simulink model "modelo_dinamico_FL"  (R2024b)
settings: Solver=ode1  StartTime=0.0  StopTime=end_time-Ts  FixedStep=Ts  RelTol=1e-3
undefined symbols (not defined in the file): du1_0, g, k11, k12, k13, k14, k21, k22, k23, k24, k31, k32, k33, k34, k41, k42, lim, M, tau, tau_phi_max, tau_phi_min, tau_psi_max, tau_psi_min, tau_theta_max, tau_theta_min, Ts, u1_0, u_max, u_min, x11_0, x1_0, x3_0, x5_0, x7_0, x9_0
libraries: eeGeneralControl x6, slident x1
settings Model: Creator=pdelr  LastModifiedBy=pdelr
settings DebuggingCC: UnconnectedInputMsg=warning  UnconnectedOutputMsg=warning  UnconnectedLineMsg=warning
settings ModelReferenceCC: EnableRefExpFcnMdlSchedulingChecks=on
settings RTWCC: GPUComputeCapability=3.5  DLArmComputeVersion=19.05

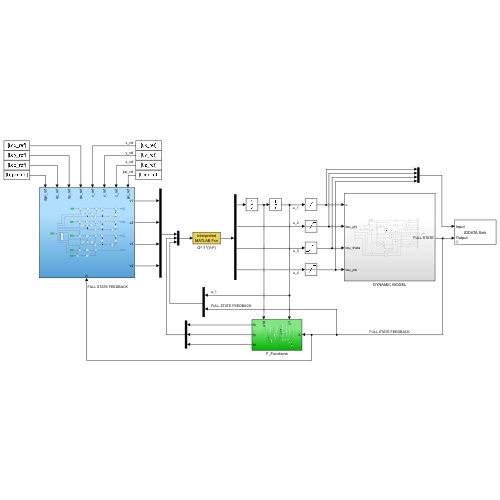
[thumbnail: Simulink's stored preview of the top-level diagram]
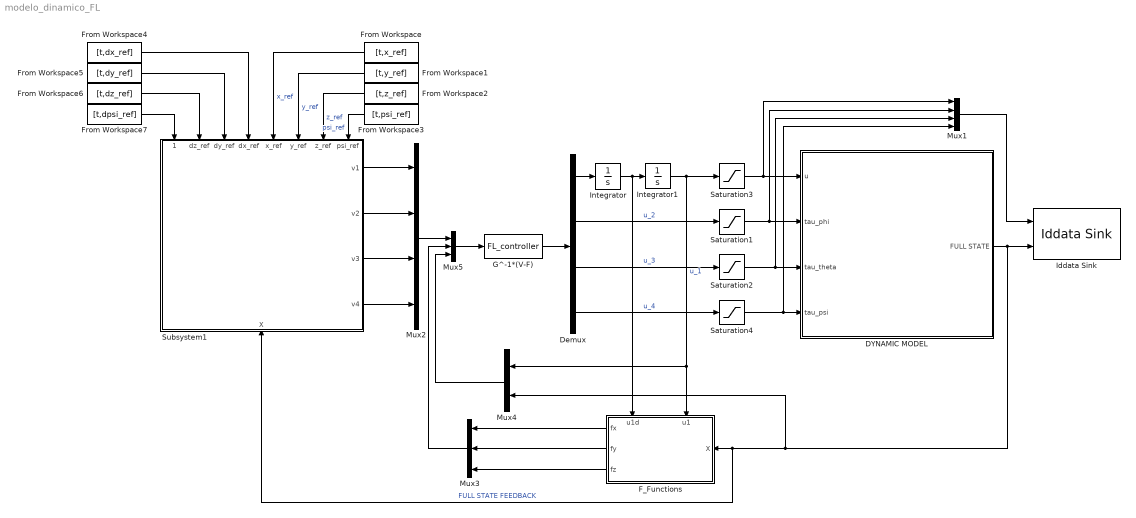
== system modelo_dinamico_FL ==
  DYNAMIC MODEL : Subsystem
  Demux : Demux
  F_Functions : Subsystem
      settings: PortSchema="{\"entries\":[{\"content\":{\"sides\":[{\"content\":{\"connectorIds\":[\"In1\"]},\"type\":\"ConnectorPlacement.EquallySpacedRectSide\",\"uuid\":\"eddb14d5-231a-4b6d-a89c-a6715b5a0e2c\"},{\"content\":{\"connectorIds\":[\"Out1\",\"Out2\",\"Out3\"],\"side\":\"RIGHT\"},\"type\":\"ConnectorPlacement.EquallySpacedRectSide\",\"uuid\":\"e1ae96f0-3fe3-4add-877e-6087d97d73d6\"},{\"content\":{\"connectorIds\":[\"In2\",\"In3\"],\"side\":\"TOP\"},\"type\":\"ConnectorPlacement.EquallySpacedRectSide\",\"uuid\":\"e0d53240-41cb-498f-be06-48178e3678e4\"},{\"content\":{\"connectorIds\":[],\"side\":\"BOTTOM\"},\"type\":\"ConnectorPlacement.EquallySpacedRectSide\",\"uuid\":\"5d003620-640e-4f1b-8c5e-2d3bbf45d64b\"}]},\"type\":\"ConnectorPlacement.EquallySpacedConnector\",\"uuid\":\"d539eae5-8b81-4451-bedc-ec98eec9f474\"}],\"packageUris\":[\"http://schema.mathworks.com/mf0/Connector/R2020b\"],\"version\":\"1.0\"}"
  From Workspace : FromWorkspace  VariableName=[t,x_ref]
  From Workspace1 : FromWorkspace  VariableName=[t,y_ref]
  From Workspace2 : FromWorkspace  VariableName=[t,z_ref]
  From Workspace3 : FromWorkspace  VariableName=[t,psi_ref]
  From Workspace4 : FromWorkspace  VariableName=[t,dx_ref]
  From Workspace5 : FromWorkspace  VariableName=[t,dy_ref]
  From Workspace6 : FromWorkspace  VariableName=[t,dz_ref]
  From Workspace7 : FromWorkspace  VariableName=[t,dpsi_ref]
  G^-1*(V-F) : MATLABFcn  MATLABFcn=FL_controller  OutputDimensions=4
  Iddata Sink : slident/Iddata Sink  datasetname=data  Ts=Ts  isu=off  isy=off
  Integrator : Integrator  InitialCondition=du1_0
  Integrator1 : Integrator  InitialCondition=u1_0  UpperSaturationLimit=lim  LowerSaturationLimit=-lim
  Mux1 : Mux
  Mux2 : Mux
  Mux3 : Mux  Inputs=3
  Mux4 : Mux  Inputs=2
  Mux5 : Mux  Inputs=3
  Saturation1 : Saturate  UpperLimit=tau_phi_max  LowerLimit=tau_phi_min
  Saturation2 : Saturate  UpperLimit=tau_theta_max  LowerLimit=tau_theta_min
  Saturation3 : Saturate  UpperLimit=u_max  LowerLimit=u_min
  Saturation4 : Saturate  UpperLimit=tau_psi_max  LowerLimit=tau_psi_min
  Subsystem1 : Subsystem
      settings: PortSchema="{\"entries\":[{\"content\":{\"sides\":[{\"content\":{\"connectorIds\":[]},\"type\":\"ConnectorPlacement.EquallySpacedRectSide\",\"uuid\":\"eddb14d5-231a-4b6d-a89c-a6715b5a0e2c\"},{\"content\":{\"connectorIds\":[\"Out1\",\"Out2\",\"Out3\",\"Out4\"],\"side\":\"RIGHT\"},\"type\":\"ConnectorPlacement.EquallySpacedRectSide\",\"uuid\":\"e1ae96f0-3fe3-4add-877e-6087d97d73d6\"},{\"content\":{\"connectorIds\":[\"In1\",\"In2\",\"In3\",\"In4\",\"In5\",\"In6\",\"In7\",\"In8\"],\"side\":\"TOP\"},\"type\":\"ConnectorPlacement.EquallySpacedRectSide\",\"uuid\":\"e0d53240-41cb-498f-be06-48178e3678e4\"},{\"content\":{\"connectorIds\":[\"In9\"],\"side\":\"BOTTOM\"},\"type\":\"ConnectorPlacement.EquallySpacedRectSide\",\"uuid\":\"99222e29-004c-4dfd-a165-743ac4cf90b4\"}]},\"type\":\"ConnectorPlacement.EquallySpacedConnector\",\"uuid\":\"d539eae5-8b81-4451-bedc-ec98eec9f474\"}],\"packageUris\":[\"http://schema.mathworks.com/mf0/Connector/R2020b\"],\"version\":\"1.0\"}"
  wires:
  Mux1/1 -> Iddata Sink/1
  Saturation3/1 -> DYNAMIC MODEL/1(u), Mux1/1
  Demux/1 -> Integrator/1
  Integrator1/1 -> Saturation3/1, Mux4/1, F_Functions/2(u1)  "u_1"
  Demux/2 -> Saturation1/1  "u_2"
  Demux/3 -> Saturation2/1  "u_3"
  Demux/4 -> Saturation4/1  "u_4"
  DYNAMIC MODEL/1(FULL STATE) -> Iddata Sink/2, F_Functions/1(X), Subsystem1/9(X), Mux4/2  "FULL STATE FEEDBACK"
  F_Functions/1(fx) -> Mux3/1
  F_Functions/2(fy) -> Mux3/2
  F_Functions/3(fz) -> Mux3/3
  Subsystem1/1(v1) -> Mux2/1
  Subsystem1/2(v2) -> Mux2/2
  Subsystem1/3(v3) -> Mux2/3
  Subsystem1/4(v4) -> Mux2/4
  Mux3/1 -> Mux5/2
  Mux4/1 -> Mux5/3
  Mux2/1 -> Mux5/1
  G^-1*(V-F)/1 -> Demux/1
  From Workspace2/1 -> Subsystem1/7(z_ref)  "z_ref"
  From Workspace3/1 -> Subsystem1/8(psi_ref)  "psi_ref"
  From Workspace/1 -> Subsystem1/5(x_ref)  "x_ref"
  From Workspace1/1 -> Subsystem1/6(y_ref)  "y_ref"
  Mux5/1 -> G^-1*(V-F)/1
  Saturation1/1 -> Mux1/2, DYNAMIC MODEL/2(tau_phi)
  Saturation4/1 -> Mux1/4, DYNAMIC MODEL/4(tau_psi)
  Integrator/1 -> F_Functions/3(u1d), Integrator1/1
  Saturation2/1 -> Mux1/3, DYNAMIC MODEL/3(tau_theta)
  From Workspace4/1 -> Subsystem1/4(dx_ref)
  From Workspace5/1 -> Subsystem1/3(dy_ref)
  From Workspace6/1 -> Subsystem1/2(dz_ref)
  From Workspace7/1 -> Subsystem1/1(dpsi_ref)

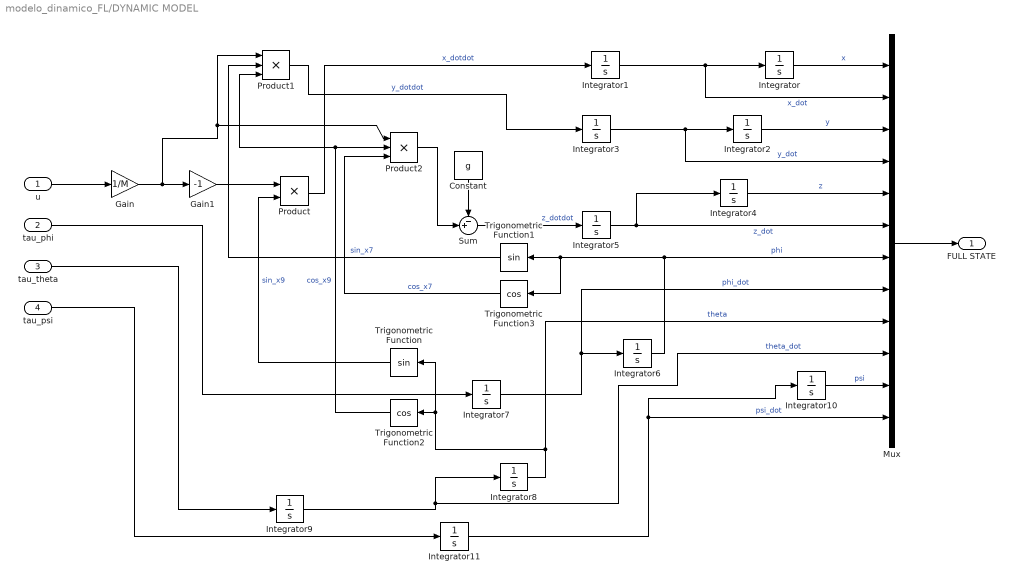
== system modelo_dinamico_FL/DYNAMIC MODEL ==
  u : Inport
  tau_phi : Inport  Port=2
  tau_theta : Inport  Port=3
  tau_psi : Inport  Port=4
  Constant : Constant  Value=g
  Gain : Gain  Gain=1/M
  Gain1 : Gain  Gain=-1
  Integrator : Integrator  InitialCondition=x1_0
  Integrator{1,3,5,7,9,11} (6 alike) : Integrator
  Integrator10 : Integrator  InitialCondition=x11_0
  Integrator2 : Integrator  InitialCondition=x3_0
  Integrator4 : Integrator  InitialCondition=x5_0
  Integrator6 : Integrator  InitialCondition=x7_0
  Integrator8 : Integrator  InitialCondition=x9_0
  Mux : Mux  Inputs=12
  Product : Product
  Product1 : Product  Inputs=3
  Product2 : Product  Inputs=3
  Sum : Sum  Inputs=-+|
  Trigonometric Function : Trigonometry
  Trigonometric Function1 : Trigonometry
  Trigonometric Function2 : Trigonometry  Operator=cos
  Trigonometric Function3 : Trigonometry  Operator=cos
  FULL STATE : Outport
  wires:
  Integrator5/1 -> Integrator4/1, Mux/6  "z_dot"
  Integrator8/1 -> Mux/9, Trigonometric Function2/1, Trigonometric Function/1  "theta"
  Integrator3/1 -> Mux/4, Integrator2/1  "y_dot"
  Integrator7/1 -> Integrator6/1, Mux/8  "phi_dot"
  Trigonometric Function3/1 -> Product2/3  "cos_x7"
  Integrator2/1 -> Mux/3  "y"
  Integrator6/1 -> Trigonometric Function3/1, Trigonometric Function1/1, Mux/7  "phi"
  Integrator9/1 -> Mux/10, Integrator8/1  "theta_dot"
  Product1/1 -> Integrator3/1  "y_dotdot"
  Product/1 -> Integrator1/1  "x_dotdot"
  Trigonometric Function/1 -> Product/2  "sin_x9"
  Integrator/1 -> Mux/1  "x"
  Trigonometric Function1/1 -> Product1/2  "sin_x7"
  Integrator4/1 -> Mux/5  "z"
  Trigonometric Function2/1 -> Product2/2, Product1/3  "cos_x9"
  Integrator11/1 -> Integrator10/1, Mux/12  "psi_dot"
  Integrator1/1 -> Mux/2, Integrator/1  "x_dot"
  Gain/1 -> Gain1/1, Product1/1, Product2/1
  Integrator10/1 -> Mux/11  "psi"
  Gain1/1 -> Product/1
  Sum/1 -> Integrator5/1  "z_dotdot"
  Product2/1 -> Sum/2
  Constant/1 -> Sum/1
  u/1 -> Gain/1
  tau_phi/1 -> Integrator7/1
  tau_psi/1 -> Integrator11/1
  tau_theta/1 -> Integrator9/1
  Mux/1 -> FULL STATE/1

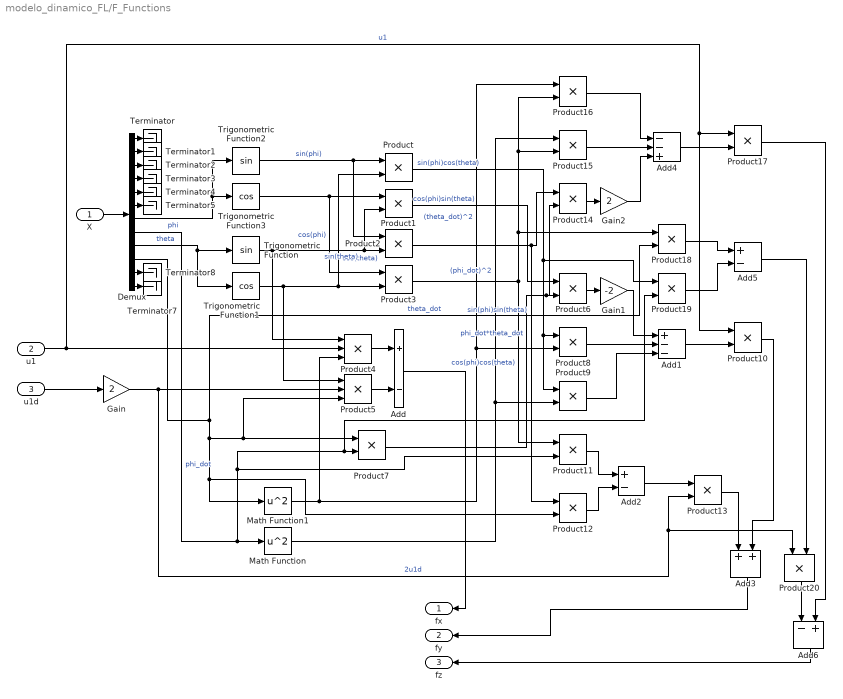
== system modelo_dinamico_FL/F_Functions ==
  X : Inport
  u1 : Inport  Port=2
  u1d : Inport  Port=3
  Add : Sum  Inputs=+-
  Add1 : Sum  Inputs=+--
  Add2 : Sum  Inputs=+-
  Add3 : Sum
  Add4 : Sum  Inputs=--+
  Add5 : Sum  Inputs=+-
  Add6 : Sum  Inputs=-+
  Demux : Demux  Outputs=12
  Gain : Gain  Gain=2
  Gain1 : Gain  Gain=-2
  Gain2 : Gain  Gain=2
  Math Function : Math  Operator=square
  Math Function1 : Math  Operator=square
  Product{,1..3,6..20} (19 alike) : Product
  Product4 : Product  Inputs=3
  Product5 : Product  Inputs=3
  Terminator{,1..5,7..8} (8 alike) : Terminator
  Trigonometric Function : Trigonometry
  Trigonometric Function1 : Trigonometry  Operator=cos
  Trigonometric Function2 : Trigonometry
  Trigonometric Function3 : Trigonometry  Operator=cos
  fx : Outport
  fy : Outport  Port=2
  fz : Outport  Port=3
  wires:
  Demux/9 -> Trigonometric Function1/1, Trigonometric Function/1  "theta"
  Add/1 -> fx/1
  Demux/7 -> Trigonometric Function2/1, Trigonometric Function3/1  "phi"
  Trigonometric Function2/1 -> Product2/1, Product/1  "sin(phi)"
  Trigonometric Function1/1 -> Product5/1, Product/2, Product3/2  "cos(theta)"
  Trigonometric Function3/1 -> Product3/1, Product1/1  "cos(phi)"
  Trigonometric Function/1 -> Product4/1, Product1/2, Product2/2  "sin(theta)"
  Product/1 -> Product19/1, Product9/1, Product8/1  "sin(phi)cos(theta)"
  Product1/1 -> Product6/1  "cos(phi)sin(theta)"
  Product2/1 -> Product14/1, Product12/1  "sin(phi)sin(theta)"
  u1d/1 -> Gain/1
  Demux/8 -> Product19/2, Product7/2, Product11/2, Math Function/1  "phi_dot"
  Demux/10 -> Math Function1/1, Product12/2, Product7/1, Product5/3, Product18/2  "theta_dot"
  u1/1 -> Product17/1, Product10/1, Product4/2  "u1"
  Math Function1/1 -> Product16/1, Product8/2, Product4/3  "(theta_dot)^2"
  Gain/1 -> Product20/1, Product13/2, Product5/2  "2u1d"
  Product5/1 -> Add/2
  Product4/1 -> Add/1
  Product7/1 -> Product14/2, Product6/2  "phi_dot*theta_dot"
  Product6/1 -> Gain1/1
  Math Function/1 -> Product15/1, Product9/2  "(phi_dot)^2"
  Gain1/1 -> Add1/1
  Product8/1 -> Add1/2
  Product9/1 -> Add1/3
  Add1/1 -> Product10/2
  Product3/1 -> Product16/2, Product15/2, Product18/1, Product11/1  "cos(phi)cos(theta)"
  Product11/1 -> Add2/1
  Product12/1 -> Add2/2
  Add2/1 -> Product13/1
  Product10/1 -> Add3/2
  Product13/1 -> Add3/1
  Add3/1 -> fy/1
  Product14/1 -> Gain2/1
  Gain2/1 -> Add4/3
  Product15/1 -> Add4/2
  Product16/1 -> Add4/1
  Add4/1 -> Product17/2
  Product18/1 -> Add5/1
  Product19/1 -> Add5/2
  Add5/1 -> Product20/2
  Product17/1 -> Add6/2
  Product20/1 -> Add6/1
  Add6/1 -> fz/1
  X/1 -> Demux/1
  Demux/1 -> Terminator/1
  Demux/2 -> Terminator1/1
  Demux/3 -> Terminator2/1
  Demux/4 -> Terminator3/1
  Demux/5 -> Terminator4/1
  Demux/6 -> Terminator5/1
  Demux/12 -> Terminator7/1
  Demux/11 -> Terminator8/1

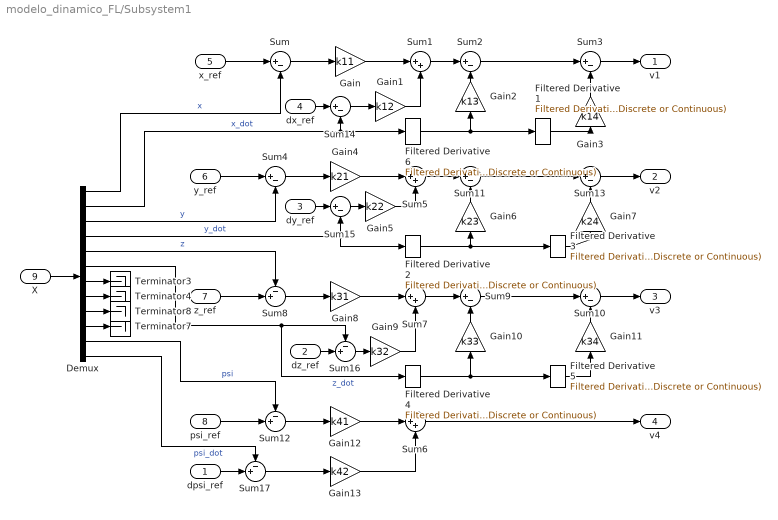
== system modelo_dinamico_FL/Subsystem1 ==
  dpsi_ref : Inport
  dz_ref : Inport  Port=2
  dy_ref : Inport  Port=3
  dx_ref : Inport  Port=4
  x_ref : Inport  Port=5
  y_ref : Inport  Port=6
  z_ref : Inport  Port=7
  psi_ref : Inport  Port=8
  X : Inport  Port=9
  Demux : Demux  Outputs=12
  Filtered Derivative {1..6} (6 alike) : eeGeneralControl/Filtered Derivative (Discrete or Continuous)  K=1  T=tau  B=lim  A=-lim  minRatio=10  init_option=Inherited from block input  x0=0  Ts=Ts
  Gain : Gain  Gain=k11
  Gain1 : Gain  Gain=k12
  Gain10 : Gain  Gain=k33
  Gain11 : Gain  Gain=k34
  Gain12 : Gain  Gain=k41
  Gain13 : Gain  Gain=k42
  Gain2 : Gain  Gain=k13
  Gain3 : Gain  Gain=k14
  Gain4 : Gain  Gain=k21
  Gain5 : Gain  Gain=k22
  Gain6 : Gain  Gain=k23
  Gain7 : Gain  Gain=k24
  Gain8 : Gain  Gain=k31
  Gain9 : Gain  Gain=k32
  Sum{,2..4,9..11,13..15} (10 alike) : Sum  Inputs=|+-
  Sum{1,5..7} (4 alike) : Sum  Inputs=|++
  Sum{8,12,16..17} (4 alike) : Sum  Inputs=-+|
  Terminator{3..4,7..8} (4 alike) : Terminator
  v1 : Outport
  v2 : Outport  Port=2
  v3 : Outport  Port=3
  v4 : Outport  Port=4
  wires:
  x_ref/1 -> Sum/1
  Demux/1 -> Sum/2  "x"
  Sum/1 -> Gain/1
  Gain/1 -> Sum1/1
  Gain1/1 -> Sum1/2
  Gain2/1 -> Sum2/2
  Sum1/1 -> Sum2/1
  Sum2/1 -> Sum3/1
  Gain3/1 -> Sum3/2
  Sum5/1 -> Sum11/1
  Sum11/1 -> Sum13/1
  Gain6/1 -> Sum11/2
  Gain4/1 -> Sum5/1
  Demux/3 -> Sum4/2  "y"
  Sum4/1 -> Gain4/1
  Gain7/1 -> Sum13/2
  y_ref/1 -> Sum4/1
  Gain5/1 -> Sum5/2
  Demux/5 -> Sum8/1  "z"
  z_ref/1 -> Sum8/2
  Demux/6 -> Filtered Derivative 4/1, Sum16/1  "z_dot"
  Gain10/1 -> Sum9/2
  Sum7/1 -> Sum9/1
  Sum9/1 -> Sum10/1
  Gain9/1 -> Sum7/2
  Gain11/1 -> Sum10/2
  Sum8/1 -> Gain8/1
  Gain8/1 -> Sum7/1
  Gain12/1 -> Sum6/1
  Gain13/1 -> Sum6/2
  Sum12/1 -> Gain12/1
  psi_ref/1 -> Sum12/2
  Demux/11 -> Sum12/1  "psi"
  X/1 -> Demux/1
  Demux/4 -> Sum15/2, Filtered Derivative 2/1  "y_dot"
  Demux/7 -> Terminator3/1
  Demux/9 -> Terminator8/1
  Demux/10 -> Terminator7/1
  Demux/8 -> Terminator4/1
  Demux/2 -> Filtered Derivative 6/1, Sum14/2  "x_dot"
  Sum14/1 -> Gain1/1
  Sum15/1 -> Gain5/1
  Sum16/1 -> Gain9/1
  Demux/12 -> Sum17/1  "psi_dot"
  Sum17/1 -> Gain13/1
  Filtered Derivative 6/1 -> Filtered Derivative 1/1, Gain2/1
  Filtered Derivative 1/1 -> Gain3/1
  Sum3/1 -> v1/1
  Sum13/1 -> v2/1
  Sum10/1 -> v3/1
  Sum6/1 -> v4/1
  Filtered Derivative 2/1 -> Filtered Derivative 3/1, Gain6/1
  Filtered Derivative 4/1 -> Filtered Derivative 5/1, Gain10/1
  Filtered Derivative 3/1 -> Gain7/1
  Filtered Derivative 5/1 -> Gain11/1
  dx_ref/1 -> Sum14/1
  dy_ref/1 -> Sum15/1
  dz_ref/1 -> Sum16/2
  dpsi_ref/1 -> Sum17/2
